simulink model "SecRwRtStFtrstIsPosChk"  (R2024b)
settings: Solver=FixedStepDiscrete  StartTime=0.0  StopTime=10.0  FixedStep=0.01  RelTol=1e-3
undefined symbols (not defined in the file or in its folder): KeSMSuSecRwStFtrstUpwdDnwdPosDelta_Val, KeSMSuSecRwStFtrstUpwdDnwdPosTolr_Val
libraries: StIsPosChkLib x9, simulink x5
settings Model: ModifiedHistory=2023.8.1 V2.0.0 CR421790 增加模式21-26  Creator=sn2xws  LastModifiedBy=sn55gm
settings SolverCC: AlgebraicLoopSolver=TrustRegion
settings DataIOCC: SaveFormat=StructureWithTime  ReturnWorkspaceOutputs=off
settings OptimizationCC: DefaultParameterBehavior=Inlined  EnhancedBackFolding=on  PassReuseOutputArgsAs=Individual arguments  ZeroExternalMemoryAtStartup=off  ZeroInternalMemoryAtStartup=off  OptimizeBlockOrder=speed  DifferentSizesBufferReuse=on  OptimizationCustomize=off  EfficientTunableParamExpr=on
settings DebuggingCC: ParameterTunabilityLossMsg=error  UnconnectedInputMsg=warning  UnconnectedOutputMsg=warning  UnconnectedLineMsg=warning  ArithmeticOperatorsInVariantConditions=warning
settings ModelReferenceCC: EnableRefExpFcnMdlSchedulingChecks=on  ModelReferenceNumInstancesAllowed=Single
settings SFSimCC: MATLABDynamicMemAlloc=off  CustomCodeUndefinedFunction=UseInterfaceOnly
settings RTWCC: Description=AUTOSAR  SystemTargetFile=autosar.tlc  GenCodeOnly=on  TemplateMakefile=ert_default_tmf  GenerateReport=on  IncludeHyperlinkInReport=on  LaunchReport=on  DataTypeReplacement=CDataTypesFixedWidth  GenerateTraceInfo=on  GenerateTraceReport=on  GenerateTraceReportSl=on  GenerateTraceReportSf=on  GenerateTraceReportEml=on  GPUComputeCapability=3.5
settings CodeAppCC: ForceParamTrailComments=on  IgnoreCustomStorageClasses=off  OperatorAnnotations=on  SimulinkDataObjDesc=on  SFDataObjDesc=on  InsertBlockDesc=on
settings STFCustomTargetCC: TargetLangStandard=C99 (ISO)  MultiwordLength=256  ParMdlRefBuildCompliant=on  CompOptLevelCompliant=on  IncludeMdlTerminateFcn=off  CombineOutputUpdateFcns=on  SuppressErrorStatus=on  ERTCustomFileBanners=on  SupportNonFinite=off  SupportComplex=off  SupportContinuousTime=off  SupportNonInlinedSFcns=off  RemoveResetFunc=on  MATLABClassNameForMDSCustomization=Simulink.SoftwareTarget.ERTCustomization  AutosarCompliant=on  UseToolchainInfoCompliant=on  LookupTableObjectStructAxisOrder=2,1,3,4,...  LUTObjectStructOrderEvenSpacing=Size,Table,Breakpoints  SystemTargetFile=autosar.tlc
settings ERTTargetCC: TargetLangStandard=C99 (ISO)  ConcurrentExecutionCompliant=off  IncludeMdlTerminateFcn=off  SuppressErrorStatus=on  SupportNonFinite=off  SupportComplex=off  ModelStepFunctionPrototypeControlCompliant=off  CPPClassGenCompliant=off  AutosarCompliant=on  LookupTableObjectStructAxisOrder=2,1,3,4,...  LUTObjectStructOrderEvenSpacing=Size,Table,Breakpoints  ERTCustomFileTemplate=example_file_process.tlc  ERTFilePackagingFormat=Compact  BooleanTrueId=TRUE  BooleanFalseId=FALSE  DynamicArrayContainerType=coder::array

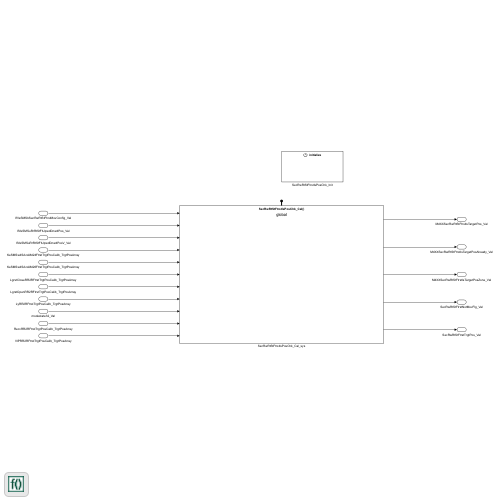
[thumbnail: Simulink's stored preview of the top-level diagram]
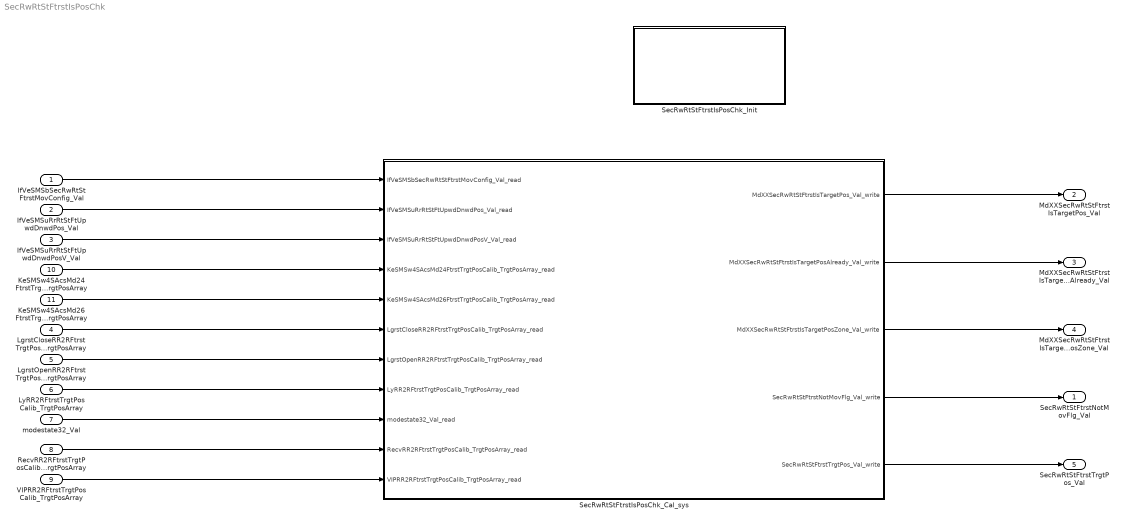
== system SecRwRtStFtrstIsPosChk ==
  IfVeSMSbSecRwRtStFtrstMovConfig_Val : Inport  OutDataTypeStr=boolean  PortDimensions=1
  IfVeSMSuRrRtStFtUpwdDnwdPos_Val : Inport  Port=2  OutDataTypeStr=uint16  PortDimensions=1
  IfVeSMSuRrRtStFtUpwdDnwdPosV_Val : Inport  Port=3  OutDataTypeStr=boolean  PortDimensions=1
  LgrstCloseRR2RFtrstTrgtPosCalib_TrgtPosArray : Inport  Description=|  Port=4  OutDataTypeStr=uint16  PortDimensions=3
      | 0:Pos
      | 1:Max
      | 2:Min
  LgrstOpenRR2RFtrstTrgtPosCalib_TrgtPosArray : Inport  Description=|  Port=5  OutDataTypeStr=uint16  PortDimensions=3
      | 0:Pos
      | 1:Max
      | 2:Min
  LyRR2RFtrstTrgtPosCalib_TrgtPosArray : Inport  Description=|  Port=6  OutDataTypeStr=uint16  PortDimensions=3
      | 0:Pos
      | 1:Max
      | 2:Min
  modestate32_Val : Inport  Port=7  OutDataTypeStr=uint32  PortDimensions=1
  RecvRR2RFtrstTrgtPosCalib_TrgtPosArray : Inport  Description=|  Port=8  OutDataTypeStr=uint16  PortDimensions=3
      | 0:Pos
      | 1:Max
      | 2:Min
  VIPRR2RFtrstTrgtPosCalib_TrgtPosArray : Inport  Description=|  Port=9  OutDataTypeStr=uint16  PortDimensions=3
      | 0:Pos
      | 1:Max
      | 2:Min
  KeSMSw4SAcsMd24FtrstTrgtPosCalib_TrgtPosArray : Inport  Description=|  Port=10  OutDataTypeStr=uint16  PortDimensions=3
      | 0:Pos
      | 1:Max
      | 2:Min
  KeSMSw4SAcsMd26FtrstTrgtPosCalib_TrgtPosArray : Inport  Description=|  Port=11  OutDataTypeStr=uint16  PortDimensions=3
      | 0:Pos
      | 1:Max
      | 2:Min
  SecRwRtStFtrstIsPosChk_Cal_sys : Subsystem
  SecRwRtStFtrstIsPosChk_Init : Subsystem
  SecRwRtStFtrstNotMovFlg_Val : Outport  OutDataTypeStr=boolean  PortDimensions=1  VectorParamsAs1DForOutWhenUnconnected=off
  MdXXSecRwRtStFtrstIsTargetPos_Val : Outport  Port=2  OutDataTypeStr=uint32  PortDimensions=1  VectorParamsAs1DForOutWhenUnconnected=off
  MdXXSecRwRtStFtrstIsTargetPosAlready_Val : Outport  Port=3  OutDataTypeStr=uint32  PortDimensions=1  VectorParamsAs1DForOutWhenUnconnected=off
  MdXXSecRwRtStFtrstIsTargetPosZone_Val : Outport  Port=4  OutDataTypeStr=uint32  PortDimensions=1  VectorParamsAs1DForOutWhenUnconnected=off
  SecRwRtStFtrstTrgtPos_Val : Outport  Port=5  OutDataTypeStr=uint16  PortDimensions=1  VectorParamsAs1DForOutWhenUnconnected=off
  wires:
  IfVeSMSbSecRwRtStFtrstMovConfig_Val/1 -> SecRwRtStFtrstIsPosChk_Cal_sys/1(IfVeSMSbSecRwRtStFtrstMovConfig_Val_read)
  IfVeSMSuRrRtStFtUpwdDnwdPos_Val/1 -> SecRwRtStFtrstIsPosChk_Cal_sys/2(IfVeSMSuRrRtStFtUpwdDnwdPos_Val_read)
  IfVeSMSuRrRtStFtUpwdDnwdPosV_Val/1 -> SecRwRtStFtrstIsPosChk_Cal_sys/3(IfVeSMSuRrRtStFtUpwdDnwdPosV_Val_read)
  LgrstCloseRR2RFtrstTrgtPosCalib_TrgtPosArray/1 -> SecRwRtStFtrstIsPosChk_Cal_sys/6(LgrstCloseRR2RFtrstTrgtPosCalib_TrgtPosArray_read)
  LgrstOpenRR2RFtrstTrgtPosCalib_TrgtPosArray/1 -> SecRwRtStFtrstIsPosChk_Cal_sys/7(LgrstOpenRR2RFtrstTrgtPosCalib_TrgtPosArray_read)
  LyRR2RFtrstTrgtPosCalib_TrgtPosArray/1 -> SecRwRtStFtrstIsPosChk_Cal_sys/8(LyRR2RFtrstTrgtPosCalib_TrgtPosArray_read)
  modestate32_Val/1 -> SecRwRtStFtrstIsPosChk_Cal_sys/9(modestate32_Val_read)
  RecvRR2RFtrstTrgtPosCalib_TrgtPosArray/1 -> SecRwRtStFtrstIsPosChk_Cal_sys/10(RecvRR2RFtrstTrgtPosCalib_TrgtPosArray_read)
  VIPRR2RFtrstTrgtPosCalib_TrgtPosArray/1 -> SecRwRtStFtrstIsPosChk_Cal_sys/11(VIPRR2RFtrstTrgtPosCalib_TrgtPosArray_read)
  SecRwRtStFtrstIsPosChk_Cal_sys/1(MdXXSecRwRtStFtrstIsTargetPos_Val_write) -> MdXXSecRwRtStFtrstIsTargetPos_Val/1
  SecRwRtStFtrstIsPosChk_Cal_sys/4(SecRwRtStFtrstNotMovFlg_Val_write) -> SecRwRtStFtrstNotMovFlg_Val/1
  SecRwRtStFtrstIsPosChk_Cal_sys/5(SecRwRtStFtrstTrgtPos_Val_write) -> SecRwRtStFtrstTrgtPos_Val/1
  KeSMSw4SAcsMd24FtrstTrgtPosCalib_TrgtPosArray/1 -> SecRwRtStFtrstIsPosChk_Cal_sys/4(KeSMSw4SAcsMd24FtrstTrgtPosCalib_TrgtPosArray_read)
  KeSMSw4SAcsMd26FtrstTrgtPosCalib_TrgtPosArray/1 -> SecRwRtStFtrstIsPosChk_Cal_sys/5(KeSMSw4SAcsMd26FtrstTrgtPosCalib_TrgtPosArray_read)
  SecRwRtStFtrstIsPosChk_Cal_sys/3(MdXXSecRwRtStFtrstIsTargetPosZone_Val_write) -> MdXXSecRwRtStFtrstIsTargetPosZone_Val/1
  SecRwRtStFtrstIsPosChk_Cal_sys/2(MdXXSecRwRtStFtrstIsTargetPosAlready_Val_write) -> MdXXSecRwRtStFtrstIsTargetPosAlready_Val/1

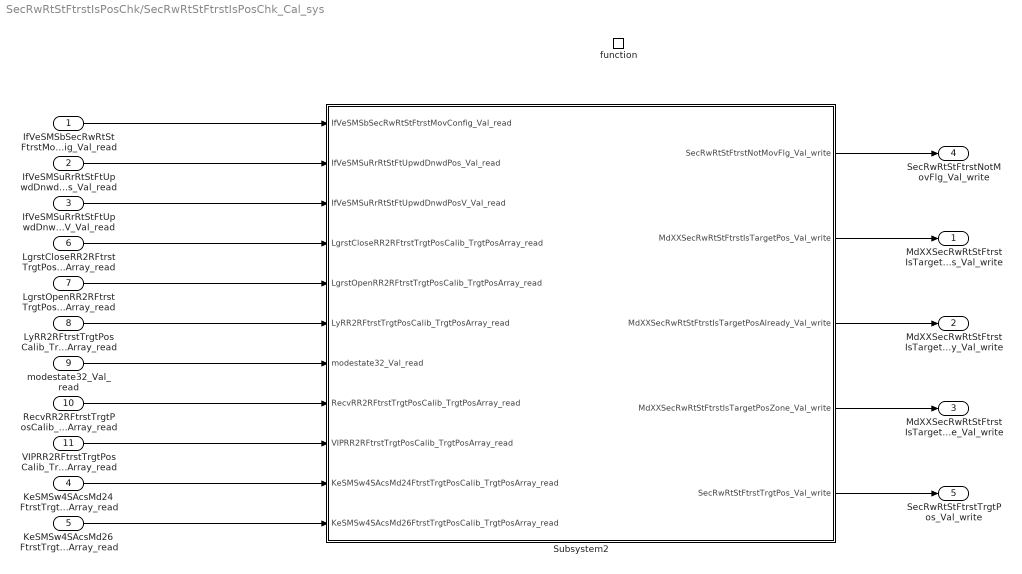
== system SecRwRtStFtrstIsPosChk/SecRwRtStFtrstIsPosChk_Cal_sys ==
  IfVeSMSbSecRwRtStFtrstMovConfig_Val_read : Inport
  IfVeSMSuRrRtStFtUpwdDnwdPos_Val_read : Inport  Port=2
  IfVeSMSuRrRtStFtUpwdDnwdPosV_Val_read : Inport  Port=3
  KeSMSw4SAcsMd24FtrstTrgtPosCalib_TrgtPosArray_read : Inport  Port=4
  KeSMSw4SAcsMd26FtrstTrgtPosCalib_TrgtPosArray_read : Inport  Port=5
  LgrstCloseRR2RFtrstTrgtPosCalib_TrgtPosArray_read : Inport  Port=6
  LgrstOpenRR2RFtrstTrgtPosCalib_TrgtPosArray_read : Inport  Port=7
  LyRR2RFtrstTrgtPosCalib_TrgtPosArray_read : Inport  Port=8
  modestate32_Val_read : Inport  Port=9
  RecvRR2RFtrstTrgtPosCalib_TrgtPosArray_read : Inport  Port=10
  VIPRR2RFtrstTrgtPosCalib_TrgtPosArray_read : Inport  Port=11
  function : TriggerPort  TriggerType=function-call  IsSimulinkFunction=on  FunctionName=SecRwRtStFtrstIsPosChk_Cal  VariantControl=(inherit)
  Subsystem2 : Subsystem
  MdXXSecRwRtStFtrstIsTargetPos_Val_write : Outport  VectorParamsAs1DForOutWhenUnconnected=off
      settings: EnsureOutportIsVirtual=on
  MdXXSecRwRtStFtrstIsTargetPosAlready_Val_write : Outport  Port=2  VectorParamsAs1DForOutWhenUnconnected=off
      settings: EnsureOutportIsVirtual=on
  MdXXSecRwRtStFtrstIsTargetPosZone_Val_write : Outport  Port=3  VectorParamsAs1DForOutWhenUnconnected=off
      settings: EnsureOutportIsVirtual=on
  SecRwRtStFtrstNotMovFlg_Val_write : Outport  Port=4  VectorParamsAs1DForOutWhenUnconnected=off
      settings: EnsureOutportIsVirtual=on
  SecRwRtStFtrstTrgtPos_Val_write : Outport  Port=5  VectorParamsAs1DForOutWhenUnconnected=off
      settings: EnsureOutportIsVirtual=on
  wires:
  LgrstCloseRR2RFtrstTrgtPosCalib_TrgtPosArray_read/1 -> Subsystem2/4(LgrstCloseRR2RFtrstTrgtPosCalib_TrgtPosArray_read)
  IfVeSMSuRrRtStFtUpwdDnwdPosV_Val_read/1 -> Subsystem2/3(IfVeSMSuRrRtStFtUpwdDnwdPosV_Val_read)
  LgrstOpenRR2RFtrstTrgtPosCalib_TrgtPosArray_read/1 -> Subsystem2/5(LgrstOpenRR2RFtrstTrgtPosCalib_TrgtPosArray_read)
  IfVeSMSuRrRtStFtUpwdDnwdPos_Val_read/1 -> Subsystem2/2(IfVeSMSuRrRtStFtUpwdDnwdPos_Val_read)
  LyRR2RFtrstTrgtPosCalib_TrgtPosArray_read/1 -> Subsystem2/6(LyRR2RFtrstTrgtPosCalib_TrgtPosArray_read)
  IfVeSMSbSecRwRtStFtrstMovConfig_Val_read/1 -> Subsystem2/1(IfVeSMSbSecRwRtStFtrstMovConfig_Val_read)
  modestate32_Val_read/1 -> Subsystem2/7(modestate32_Val_read)
  RecvRR2RFtrstTrgtPosCalib_TrgtPosArray_read/1 -> Subsystem2/8(RecvRR2RFtrstTrgtPosCalib_TrgtPosArray_read)
  VIPRR2RFtrstTrgtPosCalib_TrgtPosArray_read/1 -> Subsystem2/9(VIPRR2RFtrstTrgtPosCalib_TrgtPosArray_read)
  KeSMSw4SAcsMd24FtrstTrgtPosCalib_TrgtPosArray_read/1 -> Subsystem2/10(KeSMSw4SAcsMd24FtrstTrgtPosCalib_TrgtPosArray_read)
  KeSMSw4SAcsMd26FtrstTrgtPosCalib_TrgtPosArray_read/1 -> Subsystem2/11(KeSMSw4SAcsMd26FtrstTrgtPosCalib_TrgtPosArray_read)
  Subsystem2/1(SecRwRtStFtrstNotMovFlg_Val_write) -> SecRwRtStFtrstNotMovFlg_Val_write/1
  Subsystem2/2(MdXXSecRwRtStFtrstIsTargetPos_Val_write) -> MdXXSecRwRtStFtrstIsTargetPos_Val_write/1
  Subsystem2/3(MdXXSecRwRtStFtrstIsTargetPosAlready_Val_write) -> MdXXSecRwRtStFtrstIsTargetPosAlready_Val_write/1
  Subsystem2/4(MdXXSecRwRtStFtrstIsTargetPosZone_Val_write) -> MdXXSecRwRtStFtrstIsTargetPosZone_Val_write/1
  Subsystem2/5(SecRwRtStFtrstTrgtPos_Val_write) -> SecRwRtStFtrstTrgtPos_Val_write/1

== system SecRwRtStFtrstIsPosChk/SecRwRtStFtrstIsPosChk_Init ==
  Event Listener : EventListener  EventName=reset

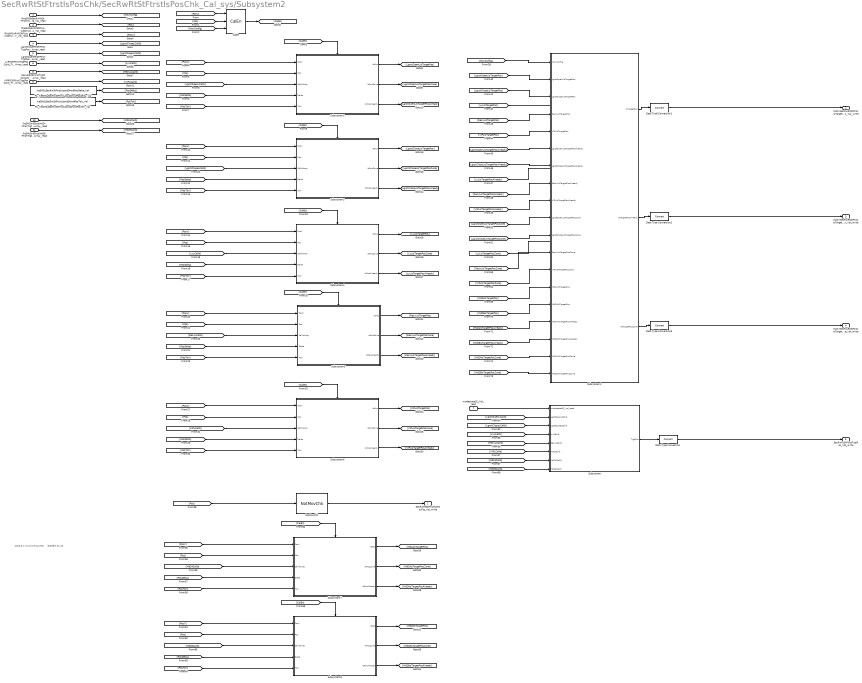
== system SecRwRtStFtrstIsPosChk/SecRwRtStFtrstIsPosChk_Cal_sys/Subsystem2 ==
  note: 2023.8.1 V2.0.0 CR421790 增加模式21-26
  IfVeSMSbSecRwRtStFtrstMovConfig_Val_read : Inport
  IfVeSMSuRrRtStFtUpwdDnwdPos_Val_read : Inport  Port=2
  IfVeSMSuRrRtStFtUpwdDnwdPosV_Val_read : Inport  Port=3
  LgrstCloseRR2RFtrstTrgtPosCalib_TrgtPosArray_read : Inport  Port=4
  LgrstOpenRR2RFtrstTrgtPosCalib_TrgtPosArray_read : Inport  Port=5
  LyRR2RFtrstTrgtPosCalib_TrgtPosArray_read : Inport  Port=6
  modestate32_Val_read : Inport  Port=7
  RecvRR2RFtrstTrgtPosCalib_TrgtPosArray_read : Inport  Port=8
  VIPRR2RFtrstTrgtPosCalib_TrgtPosArray_read : Inport  Port=9
  KeSMSw4SAcsMd24FtrstTrgtPosCalib_TrgtPosArray_read : Inport  Port=10
  KeSMSw4SAcsMd26FtrstTrgtPosCalib_TrgtPosArray_read : Inport  Port=11
  CalEn : StIsPosChkLib/CalEn  SystemSampleTime=-1  VariantActivationTime=update diagram  AllowFlexibleInterface=on  Latency=0  AutoFrameSizeCalculation=off
  Data Type Conversion{,1..3} (4 alike) : DataTypeConversion  SaturateOnIntegerOverflow=off  RndMeth=Floor
  NotMovChk : StIsPosChkLib/NotMovChk  SystemSampleTime=-1  VariantActivationTime=update diagram  AllowFlexibleInterface=on  Latency=0  AutoFrameSizeCalculation=off
  PA_KeSMSuSecRwStFtrstUpwdDnwdPosDelta_Val : Constant  Value=KeSMSuSecRwStFtrstUpwdDnwdPosDelta_Val
  PA_KeSMSuSecRwStFtrstUpwdDnwdPosTolr_Val : Constant  Value=KeSMSuSecRwStFtrstUpwdDnwdPosTolr_Val
  Subsystem : Subsystem
  Subsystem1 : Subsystem
  Subsystem2 : Subsystem
  Subsystem3 : Subsystem
  Subsystem4 : Subsystem
  Subsystem5 : Subsystem
  Subsystem6 : Subsystem
  Subsystem7 : Subsystem
  Subsystem8 : Subsystem
  SecRwRtStFtrstNotMovFlg_Val_write : Outport  VectorParamsAs1DForOutWhenUnconnected=off
      settings: EnsureOutportIsVirtual=on
  MdXXSecRwRtStFtrstIsTargetPos_Val_write : Outport  Port=2  VectorParamsAs1DForOutWhenUnconnected=off
      settings: EnsureOutportIsVirtual=on
  MdXXSecRwRtStFtrstIsTargetPosAlready_Val_write : Outport  Port=3  VectorParamsAs1DForOutWhenUnconnected=off
      settings: EnsureOutportIsVirtual=on
  MdXXSecRwRtStFtrstIsTargetPosZone_Val_write : Outport  Port=4  VectorParamsAs1DForOutWhenUnconnected=off
      settings: EnsureOutportIsVirtual=on
  SecRwRtStFtrstTrgtPos_Val_write : Outport  Port=5  VectorParamsAs1DForOutWhenUnconnected=off
      settings: EnsureOutportIsVirtual=on
  wires:
  VIPRR2RFtrstTrgtPosCalib_TrgtPosArray_read/1 -> [VIPLCalib]
  Subsystem2/3(IsPosAlready) -> [LgrstOpenLIsTargetPosAlready]
  IfVeSMSuRrRtStFtUpwdDnwdPosV_Val_read/1 -> [PosV]
  Subsystem4/1(IsPos) -> [LyLIsTargetPos]
  IfVeSMSbSecRwRtStFtrstMovConfig_Val_read/1 -> [MovConfig]
  [CalEn] -> Subsystem5/Enable
  LgrstCloseRR2RFtrstTrgtPosCalib_TrgtPosArray_read/1 -> [LgrstCloseLCalib]
  [Pos] -> Subsystem5/2(Pos)
  IfVeSMSuRrRtStFtUpwdDnwdPos_Val_read/1 -> [Pos]
  [RecvLIsTargetPos] -> Subsystem1/4(RecvLIsTargetPos)
  [LgrstCloseLCalib] -> Subsystem/3(LgrstCloseLCalib)
  [LyLCalib] -> Subsystem/4(LyLCalib)
  [Pos] -> NotMovChk/1
  [Pos] -> Subsystem4/2(Pos)
  [PosTolr] -> Subsystem3/5(Tolr)
  PA_KeSMSuSecRwStFtrstUpwdDnwdPosTolr_Val/1 -> [PosTolr]
  [LgrstCloseLIsTargetPos] -> Subsystem1/3(LgrstCloseLIsTargetPos)
  Subsystem6/2(IsPosZone) -> [VIPLIsTargetPosZone]
  [LgrstOpenLCalib] -> Subsystem/2(LgrstOpenLCalib)
  [RecvLIsTargetPosAlready] -> Subsystem1/8(RecvLIsTargetPosAlready)
  [PosDelta] -> Subsystem4/4(Delta)
  Subsystem1/1(IsTargetPos) -> Data Type Conversion1/1
  PA_KeSMSuSecRwStFtrstUpwdDnwdPosDelta_Val/1 -> [PosDelta]
  Subsystem1/2(IsTargetPosAlready) -> Data Type Conversion2/1
  Subsystem6/3(IsPosAlready) -> [VIPLIsTargetPosAlready]
  [PosV] -> CalEn/1
  RecvRR2RFtrstTrgtPosCalib_TrgtPosArray_read/1 -> [RecvLCalib]
  [LgrstCloseLIsTargetPosZone] -> Subsystem1/11(LgrstCloseLIsTargetPosZone)
  [PosV] -> Subsystem2/1(PosV)
  [PosV] -> Subsystem6/1(PosV)
  [PosDelta] -> Subsystem3/4(Delta)
  LyRR2RFtrstTrgtPosCalib_TrgtPosArray_read/1 -> [LyLCalib]
  [RecvLIsTargetPosZone] -> Subsystem1/12(RecvLIsTargetPosZone)
  [LyLIsTargetPos] -> ?
  Data Type Conversion/1 -> SecRwRtStFtrstTrgtPos_Val_write/1
  [LyLIsTargetPosAlready] -> ?
  [MovConfig] -> Subsystem1/1(MovConfig)
  Data Type Conversion3/1 -> MdXXSecRwRtStFtrstIsTargetPosZone_Val_write/1
  [PosDelta] -> Subsystem6/4(Delta)
  [VIPLIsTargetPos] -> Subsystem1/5(VIPLIsTargetPos)
  [VIPLIsTargetPosAlready] -> Subsystem1/9(VIPLIsTargetPosAlready)
  Subsystem5/3(IsPosAlready) -> [RecvLIsTargetPosAlready]
  Subsystem4/2(IsPosZone) -> [LyLIsTargetPosZone]
  [RecvLCalib] -> Subsystem/5(RecvLCalib)
  Subsystem1/3(IsTargetPosZone) -> Data Type Conversion3/1
  Subsystem6/1(IsPos) -> [VIPLIsTargetPos]
  [VIPLIsTargetPosZone] -> Subsystem1/13(VIPLIsTargetPosZone)
  [LgrstOpenLIsTargetPos] -> Subsystem1/2(LgrstOpenLIsTargetPos)
  Subsystem/1(TrgtPos) -> Data Type Conversion/1
  [PosDelta] -> Subsystem5/4(Delta)
  [CalEn] -> Subsystem4/Enable
  Data Type Conversion2/1 -> MdXXSecRwRtStFtrstIsTargetPosAlready_Val_write/1
  Data Type Conversion1/1 -> MdXXSecRwRtStFtrstIsTargetPos_Val_write/1
  [Pos] -> Subsystem2/2(Pos)
  [CalEn] -> Subsystem3/Enable
  [LyLCalib] -> Subsystem4/3(CalibArray)
  [CalEn] -> Subsystem6/Enable
  [CalEn] -> Subsystem2/Enable
  [LgrstOpenLIsTargetPosAlready] -> Subsystem1/6(LgrstOpenLIsTargetPosAlready)
  [PosTolr] -> Subsystem2/5(Tolr)
  [PosV] -> Subsystem5/1(PosV)
  [MovConfig] -> CalEn/3
  Subsystem2/1(IsPos) -> [LgrstOpenLIsTargetPos]
  LgrstOpenRR2RFtrstTrgtPosCalib_TrgtPosArray_read/1 -> [LgrstOpenLCalib]
  Subsystem3/2(IsPosZone) -> [LgrstCloseLIsTargetPosZone]
  [Pos] -> CalEn/2
  [PosTolr] -> Subsystem4/5(Tolr)
  [LgrstOpenLIsTargetPosZone] -> Subsystem1/10(LgrstOpenLIsTargetPosZone)
  [LyLIsTargetPosZone] -> ?
  [PosDelta] -> Subsystem2/4(Delta)
  [LgrstCloseLIsTargetPosAlready] -> Subsystem1/7(LgrstCloseLIsTargetPosAlready)
  Subsystem3/1(IsPos) -> [LgrstCloseLIsTargetPos]
  [RecvLCalib] -> Subsystem5/3(CalibArray)
  [Pos] -> Subsystem6/2(Pos)
  [PosV] -> Subsystem3/1(PosV)
  Subsystem4/3(IsPosAlready) -> [LyLIsTargetPosAlready]
  [PosTolr] -> Subsystem6/5(Tolr)
  CalEn/1 -> [CalEn]
  [PosTolr] -> Subsystem5/5(Tolr)
  [VIPLCalib] -> Subsystem6/3(CalibArray)
  Subsystem2/2(IsPosZone) -> [LgrstOpenLIsTargetPosZone]
  Subsystem5/2(IsPosZone) -> [RecvLIsTargetPosZone]
  [PosV] -> Subsystem4/1(PosV)
  [Pos] -> Subsystem3/2(Pos)
  Subsystem3/3(IsPosAlready) -> [LgrstCloseLIsTargetPosAlready]
  Subsystem5/1(IsPos) -> [RecvLIsTargetPos]
  modestate32_Val_read/1 -> Subsystem/1(modestate32_Val_read)
  [VIPLCalib] -> Subsystem/6(VIPLCalib)
  NotMovChk/1 -> SecRwRtStFtrstNotMovFlg_Val_write/1
  KeSMSw4SAcsMd24FtrstTrgtPosCalib_TrgtPosArray_read/1 -> [Md24Calib]
  KeSMSw4SAcsMd26FtrstTrgtPosCalib_TrgtPosArray_read/1 -> [Md26Calib]
  [Md24Calib] -> Subsystem7/3(CalibArray)
  [PosTolr] -> Subsystem7/5(Tolr)
  [Pos] -> Subsystem7/2(Pos)
  [CalEn] -> Subsystem7/Enable
  Subsystem7/1(IsPos) -> [Md24IsTargetPos]
  [PosDelta] -> Subsystem7/4(Delta)
  [PosV] -> Subsystem7/1(PosV)
  Subsystem7/3(IsPosAlready) -> [Md24IsTargetPosAlready]
  Subsystem7/2(IsPosZone) -> [Md24IsTargetPosZone]
  Subsystem8/2(IsPosZone) -> [Md26IsTargetPosZone]
  Subsystem8/3(IsPosAlready) -> [Md26IsTargetPosAlready]
  [PosV] -> Subsystem8/1(PosV)
  [PosDelta] -> Subsystem8/4(Delta)
  Subsystem8/1(IsPos) -> [Md26IsTargetPos]
  [CalEn] -> Subsystem8/Enable
  [Pos] -> Subsystem8/2(Pos)
  [PosTolr] -> Subsystem8/5(Tolr)
  [Md26Calib] -> Subsystem8/3(CalibArray)
  [Md24Calib] -> Subsystem/7(Md24Calib)
  [Md26Calib] -> Subsystem/8(Md26Calib)
  [Md24IsTargetPos] -> Subsystem1/14(Md24IsTargetPos)
  [Md26IsTargetPos] -> Subsystem1/15(Md26IsTargetPos)
  [Md24IsTargetPosAlready] -> Subsystem1/16(Md24IsTargetPosAlready)
  [Md26IsTargetPosAlready] -> Subsystem1/17(Md26IsTargetPosAlready)
  [Md26IsTargetPosZone] -> Subsystem1/19(Md26IsTargetPosZone)
  [Md24IsTargetPosZone] -> Subsystem1/18(Md24IsTargetPosZone)
  [LgrstOpenLCalib] -> Subsystem2/3(CalibArray)
  [LgrstCloseLCalib] -> Subsystem3/3(CalibArray)

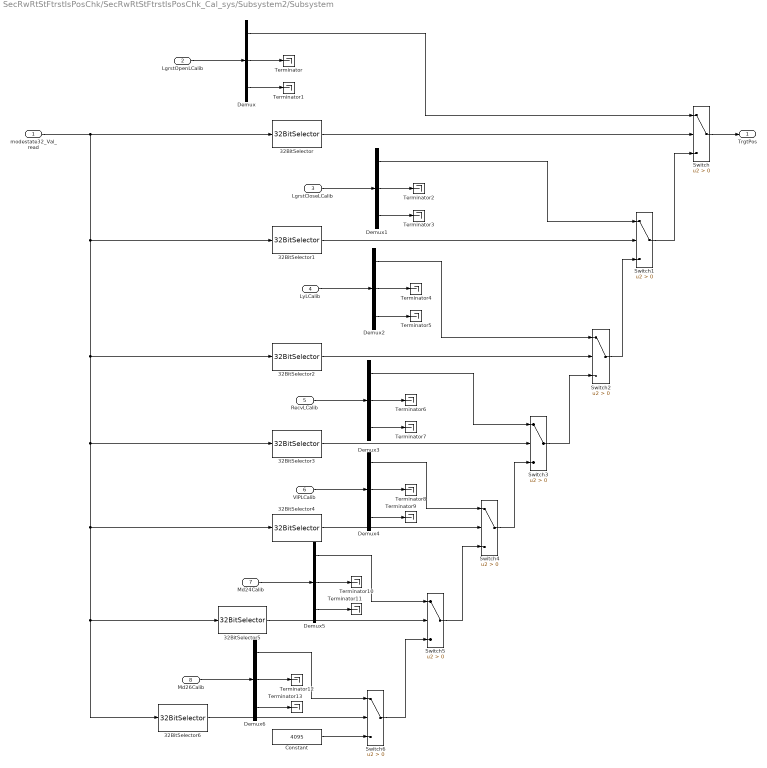
== system SecRwRtStFtrstIsPosChk/SecRwRtStFtrstIsPosChk_Cal_sys/Subsystem2/Subsystem ==
  modestate32_Val_read : Inport
  LgrstOpenLCalib : Inport  Port=2
  LgrstCloseLCalib : Inport  Port=3
  LyLCalib : Inport  Port=4
  RecvLCalib : Inport  Port=5
  VIPLCalib : Inport  Port=6
  Md24Calib : Inport  Port=7
  Md26Calib : Inport  Port=8
  32BitSelector : StIsPosChkLib/32BitSelector  BitNum=17
  32BitSelector1 : StIsPosChkLib/32BitSelector  BitNum=18
  32BitSelector2 : StIsPosChkLib/32BitSelector  BitNum=14
  32BitSelector3 : StIsPosChkLib/32BitSelector  BitNum=12
  32BitSelector4 : StIsPosChkLib/32BitSelector  BitNum=11
  32BitSelector5 : StIsPosChkLib/32BitSelector  BitNum=23
  32BitSelector6 : StIsPosChkLib/32BitSelector  BitNum=25
  Constant : Constant  Value=4095  OutDataTypeStr=uint16
  Demux{,1..6} (7 alike) : Demux  Outputs=3
  Switch{,1..6} (7 alike) : Switch  Criteria=u2 > Threshold  SaturateOnIntegerOverflow=off  InputSameDT=off
  Terminator{,1..13} (14 alike) : Terminator
  TrgtPos : Outport  VectorParamsAs1DForOutWhenUnconnected=off
      settings: EnsureOutportIsVirtual=on
  wires:
  32BitSelector/1 -> Switch/2
  modestate32_Val_read/1 -> 32BitSelector/1, 32BitSelector1/1, 32BitSelector2/1, 32BitSelector3/1, 32BitSelector6/1, 32BitSelector5/1, 32BitSelector4/1
  Demux/1 -> Switch/1
  Demux/3 -> Terminator1/1
  Demux/2 -> Terminator/1
  LgrstOpenLCalib/1 -> Demux/1
  LgrstCloseLCalib/1 -> Demux1/1
  Demux1/2 -> Terminator2/1
  Demux1/3 -> Terminator3/1
  Demux1/1 -> Switch1/1
  Switch/1 -> TrgtPos/1
  Switch1/1 -> Switch/3
  32BitSelector1/1 -> Switch1/2
  Switch2/1 -> Switch1/3
  Switch3/1 -> Switch2/3
  Switch4/1 -> Switch3/3
  32BitSelector2/1 -> Switch2/2
  32BitSelector3/1 -> Switch3/2
  32BitSelector4/1 -> Switch4/2
  Demux2/1 -> Switch2/1
  Demux2/3 -> Terminator5/1
  Demux2/2 -> Terminator4/1
  LyLCalib/1 -> Demux2/1
  RecvLCalib/1 -> Demux3/1
  Demux3/2 -> Terminator6/1
  Demux3/3 -> Terminator7/1
  Demux3/1 -> Switch3/1
  Demux4/1 -> Switch4/1
  Demux4/3 -> Terminator9/1
  Demux4/2 -> Terminator8/1
  VIPLCalib/1 -> Demux4/1
  Md24Calib/1 -> Demux5/1
  Demux5/2 -> Terminator10/1
  Demux5/3 -> Terminator11/1
  Demux5/1 -> Switch5/1
  32BitSelector5/1 -> Switch5/2
  Switch5/1 -> Switch4/3
  Switch6/1 -> Switch5/3
  32BitSelector6/1 -> Switch6/2
  Demux6/1 -> Switch6/1
  Demux6/3 -> Terminator13/1
  Demux6/2 -> Terminator12/1
  Md26Calib/1 -> Demux6/1
  Constant/1 -> Switch6/3

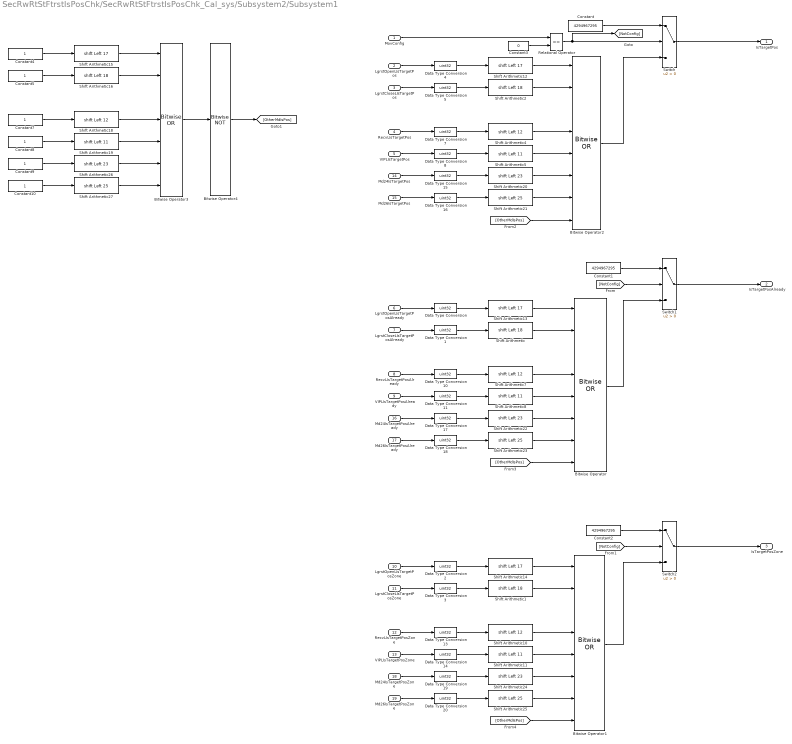
== system SecRwRtStFtrstIsPosChk/SecRwRtStFtrstIsPosChk_Cal_sys/Subsystem2/Subsystem1 ==
  MovConfig : Inport
  LgrstOpenLIsTargetPos : Inport  Port=2
  LgrstCloseLIsTargetPos : Inport  Port=3
  RecvLIsTargetPos : Inport  Port=4
  VIPLIsTargetPos : Inport  Port=5
  LgrstOpenLIsTargetPosAlready : Inport  Port=6
  LgrstCloseLIsTargetPosAlready : Inport  Port=7
  RecvLIsTargetPosAlready : Inport  Port=8
  VIPLIsTargetPosAlready : Inport  Port=9
  LgrstOpenLIsTargetPosZone : Inport  Port=10
  LgrstCloseLIsTargetPosZone : Inport  Port=11
  RecvLIsTargetPosZone : Inport  Port=12
  VIPLIsTargetPosZone : Inport  Port=13
  Md24IsTargetPos : Inport  Port=14
  Md26IsTargetPos : Inport  Port=15
  Md24IsTargetPosAlready : Inport  Port=16
  Md26IsTargetPosAlready : Inport  Port=17
  Md24IsTargetPosZone : Inport  Port=18
  Md26IsTargetPosZone : Inport  Port=19
  Bitwise Operator : simulink/Logic and Bit Operations/Bitwise Operator  logicop=OR  UseBitMask=off  NumInputPorts=8  BitMask=bin2dec('11011001')  BitMaskRealWorld=Stored Integer
  Bitwise Operator1 : simulink/Logic and Bit Operations/Bitwise Operator  logicop=OR  UseBitMask=off  NumInputPorts=8  BitMask=bin2dec('11011001')  BitMaskRealWorld=Stored Integer
  Bitwise Operator2 : simulink/Logic and Bit Operations/Bitwise Operator  logicop=OR  UseBitMask=off  NumInputPorts=8  BitMask=bin2dec('11011001')  BitMaskRealWorld=Stored Integer
  Bitwise Operator3 : simulink/Logic and Bit Operations/Bitwise Operator  logicop=OR  UseBitMask=off  NumInputPorts=7  BitMask=bin2dec('11011001')  BitMaskRealWorld=Stored Integer
  Bitwise Operator4 : simulink/Logic and Bit Operations/Bitwise Operator  logicop=NOT  UseBitMask=off  BitMask=bin2dec('11011001')  BitMaskRealWorld=Stored Integer
  Constant : Constant  Value=4294967295  OutDataTypeStr=uint32
  Constant1 : Constant  Value=4294967295  OutDataTypeStr=uint32
  Constant{4..5,7..10} (6 alike) : Constant  OutDataTypeStr=uint32
  Constant2 : Constant  Value=4294967295  OutDataTypeStr=uint32
  Constant3 : Constant  Value=0  OutDataTypeStr=uint8
  Data Type Conversion{,1..5,7..8,10..11,13..20} (18 alike) : DataTypeConversion  OutDataTypeStr=uint32  SaturateOnIntegerOverflow=off  RndMeth=Floor
  Relational Operator : RelationalOperator  Operator===  OutDataTypeStr=boolean  RndMeth=Simplest  InputSameDT=off
  Shift Arithmetic{,1..2,16} (4 alike) : ArithShift  BitShiftNumber=18  BitShiftDirection=Left
  Shift Arithmetic{4,7,10,18} (4 alike) : ArithShift  BitShiftNumber=12  BitShiftDirection=Left
  Shift Arithmetic{5,8,11,19} (4 alike) : ArithShift  BitShiftNumber=11  BitShiftDirection=Left
  Shift Arithmetic{12..15} (4 alike) : ArithShift  BitShiftNumber=17  BitShiftDirection=Left
  Shift Arithmetic{20,22,24,26} (4 alike) : ArithShift  BitShiftNumber=23  BitShiftDirection=Left
  Shift Arithmetic{21,23,25,27} (4 alike) : ArithShift  BitShiftNumber=25  BitShiftDirection=Left
  Switch : Switch  Criteria=u2 > Threshold  SaturateOnIntegerOverflow=off  InputSameDT=off
  Switch1 : Switch  Criteria=u2 > Threshold  SaturateOnIntegerOverflow=off  InputSameDT=off
  Switch2 : Switch  Criteria=u2 > Threshold  SaturateOnIntegerOverflow=off  InputSameDT=off
  IsTargetPos : Outport  VectorParamsAs1DForOutWhenUnconnected=off
      settings: EnsureOutportIsVirtual=on
  IsTargetPosAlready : Outport  Port=2  VectorParamsAs1DForOutWhenUnconnected=off
      settings: EnsureOutportIsVirtual=on
  IsTargetPosZone : Outport  Port=3  VectorParamsAs1DForOutWhenUnconnected=off
      settings: EnsureOutportIsVirtual=on
  wires:
  Constant3/1 -> Relational Operator/2
  Constant/1 -> Switch/1
  Relational Operator/1 -> [NotConfig], Switch/2
  MovConfig/1 -> Relational Operator/1
  Switch/1 -> IsTargetPos/1
  [NotConfig] -> Switch1/2
  Constant1/1 -> Switch1/1
  Switch1/1 -> IsTargetPosAlready/1
  Switch2/1 -> IsTargetPosZone/1
  Constant2/1 -> Switch2/1
  [NotConfig] -> Switch2/2
  Data Type Conversion1/1 -> Shift Arithmetic/1
  Data Type Conversion/1 -> Shift Arithmetic13/1
  Shift Arithmetic/1 -> Bitwise Operator/2
  Shift Arithmetic1/1 -> Bitwise Operator1/2
  Data Type Conversion2/1 -> Shift Arithmetic14/1
  Data Type Conversion3/1 -> Shift Arithmetic1/1
  Bitwise Operator1/1 -> Switch2/3
  Bitwise Operator/1 -> Switch1/3
  Shift Arithmetic2/1 -> Bitwise Operator2/2
  Data Type Conversion4/1 -> Shift Arithmetic12/1
  Data Type Conversion5/1 -> Shift Arithmetic2/1
  Bitwise Operator2/1 -> Switch/3
  LgrstOpenLIsTargetPos/1 -> Data Type Conversion4/1
  LgrstCloseLIsTargetPos/1 -> Data Type Conversion5/1
  LgrstCloseLIsTargetPosZone/1 -> Data Type Conversion3/1
  LgrstOpenLIsTargetPosZone/1 -> Data Type Conversion2/1
  LgrstCloseLIsTargetPosAlready/1 -> Data Type Conversion1/1
  LgrstOpenLIsTargetPosAlready/1 -> Data Type Conversion/1
  Shift Arithmetic4/1 -> Bitwise Operator2/4
  Shift Arithmetic5/1 -> Bitwise Operator2/5
  Data Type Conversion7/1 -> Shift Arithmetic4/1
  Data Type Conversion8/1 -> Shift Arithmetic5/1
  RecvLIsTargetPos/1 -> Data Type Conversion7/1
  VIPLIsTargetPos/1 -> Data Type Conversion8/1
  VIPLIsTargetPosAlready/1 -> Data Type Conversion11/1
  RecvLIsTargetPosAlready/1 -> Data Type Conversion10/1
  Data Type Conversion11/1 -> Shift Arithmetic8/1
  Data Type Conversion10/1 -> Shift Arithmetic7/1
  Shift Arithmetic8/1 -> Bitwise Operator/5
  Shift Arithmetic7/1 -> Bitwise Operator/4
  Data Type Conversion14/1 -> Shift Arithmetic11/1
  Data Type Conversion13/1 -> Shift Arithmetic10/1
  VIPLIsTargetPosZone/1 -> Data Type Conversion14/1
  Shift Arithmetic10/1 -> Bitwise Operator1/4
  RecvLIsTargetPosZone/1 -> Data Type Conversion13/1
  Shift Arithmetic11/1 -> Bitwise Operator1/5
  Shift Arithmetic12/1 -> Bitwise Operator2/1
  Shift Arithmetic13/1 -> Bitwise Operator/1
  Shift Arithmetic14/1 -> Bitwise Operator1/1
  Shift Arithmetic15/1 -> Bitwise Operator3/1
  Constant8/1 -> Shift Arithmetic19/1
  Constant7/1 -> Shift Arithmetic18/1
  Shift Arithmetic19/1 -> Bitwise Operator3/5
  Shift Arithmetic18/1 -> Bitwise Operator3/4
  Constant5/1 -> Shift Arithmetic16/1
  Constant4/1 -> Shift Arithmetic15/1
  Shift Arithmetic16/1 -> Bitwise Operator3/2
  Bitwise Operator3/1 -> Bitwise Operator4/1
  Bitwise Operator4/1 -> [OtherMdIsPos]
  [OtherMdIsPos] -> Bitwise Operator2/8
  Md24IsTargetPos/1 -> Data Type Conversion15/1
  Data Type Conversion15/1 -> Shift Arithmetic20/1
  Shift Arithmetic20/1 -> Bitwise Operator2/6
  Shift Arithmetic21/1 -> Bitwise Operator2/7
  Data Type Conversion16/1 -> Shift Arithmetic21/1
  Md26IsTargetPos/1 -> Data Type Conversion16/1
  [OtherMdIsPos] -> Bitwise Operator/8
  Shift Arithmetic22/1 -> Bitwise Operator/6
  Data Type Conversion17/1 -> Shift Arithmetic22/1
  Md24IsTargetPosAlready/1 -> Data Type Conversion17/1
  Md26IsTargetPosAlready/1 -> Data Type Conversion18/1
  Data Type Conversion18/1 -> Shift Arithmetic23/1
  Shift Arithmetic23/1 -> Bitwise Operator/7
  [OtherMdIsPos] -> Bitwise Operator1/8
  Shift Arithmetic24/1 -> Bitwise Operator1/6
  Md24IsTargetPosZone/1 -> Data Type Conversion19/1
  Data Type Conversion19/1 -> Shift Arithmetic24/1
  Data Type Conversion20/1 -> Shift Arithmetic25/1
  Md26IsTargetPosZone/1 -> Data Type Conversion20/1
  Shift Arithmetic25/1 -> Bitwise Operator1/7
  Shift Arithmetic26/1 -> Bitwise Operator3/6
  Constant9/1 -> Shift Arithmetic26/1
  Constant10/1 -> Shift Arithmetic27/1
  Shift Arithmetic27/1 -> Bitwise Operator3/7

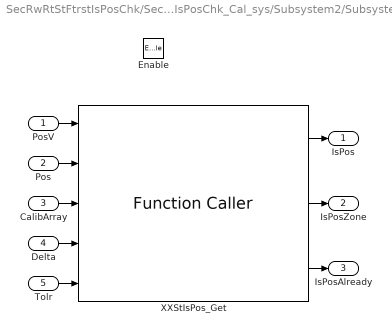
== system SecRwRtStFtrstIsPosChk/SecRwRtStFtrstIsPosChk_Cal_sys/Subsystem2/Subsystem2 ==
  PosV : Inport
  Pos : Inport  Port=2
  CalibArray : Inport  Port=3
  Delta : Inport  Port=4
  Tolr : Inport  Port=5
  Enable : EnablePort
  XXStIsPos_Get : FunctionCaller  FunctionPrototype=[IsPos,IsPosZone,IsPosAlready] = XXStIsPos_Get(PosV,Pos,CalibArray,Delta,Tolr)  InputArgumentSpecifications=boolean(true), uint16(1), uint16([1;1;1]), uint16(1), uint16(1)  OutputArgumentSpecifications=boolean(true), boolean(true), boolean(true)
  IsPos : Outport  VectorParamsAs1DForOutWhenUnconnected=off
  IsPosZone : Outport  Port=2  VectorParamsAs1DForOutWhenUnconnected=off
  IsPosAlready : Outport  Port=3  VectorParamsAs1DForOutWhenUnconnected=off
  wires:
  Delta/1 -> XXStIsPos_Get/4
  Tolr/1 -> XXStIsPos_Get/5
  XXStIsPos_Get/3 -> IsPosAlready/1
  XXStIsPos_Get/2 -> IsPosZone/1
  PosV/1 -> XXStIsPos_Get/1
  Pos/1 -> XXStIsPos_Get/2
  CalibArray/1 -> XXStIsPos_Get/3
  XXStIsPos_Get/1 -> IsPos/1

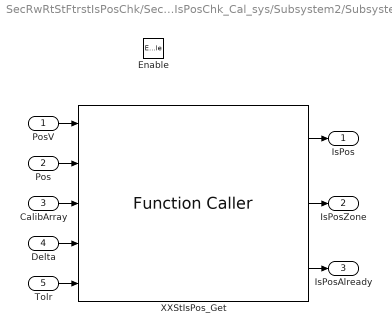
== system SecRwRtStFtrstIsPosChk/SecRwRtStFtrstIsPosChk_Cal_sys/Subsystem2/Subsystem3 ==
  PosV : Inport
  Pos : Inport  Port=2
  CalibArray : Inport  Port=3
  Delta : Inport  Port=4
  Tolr : Inport  Port=5
  Enable : EnablePort
  XXStIsPos_Get : FunctionCaller  FunctionPrototype=[IsPos,IsPosZone,IsPosAlready] = XXStIsPos_Get(PosV,Pos,CalibArray,Delta,Tolr)  InputArgumentSpecifications=boolean(true), uint16(1), uint16([1;1;1]), uint16(1), uint16(1)  OutputArgumentSpecifications=boolean(true), boolean(true), boolean(true)
  IsPos : Outport  VectorParamsAs1DForOutWhenUnconnected=off
  IsPosZone : Outport  Port=2  VectorParamsAs1DForOutWhenUnconnected=off
  IsPosAlready : Outport  Port=3  VectorParamsAs1DForOutWhenUnconnected=off
  wires:
  XXStIsPos_Get/1 -> IsPos/1
  CalibArray/1 -> XXStIsPos_Get/3
  Pos/1 -> XXStIsPos_Get/2
  PosV/1 -> XXStIsPos_Get/1
  XXStIsPos_Get/2 -> IsPosZone/1
  XXStIsPos_Get/3 -> IsPosAlready/1
  Tolr/1 -> XXStIsPos_Get/5
  Delta/1 -> XXStIsPos_Get/4

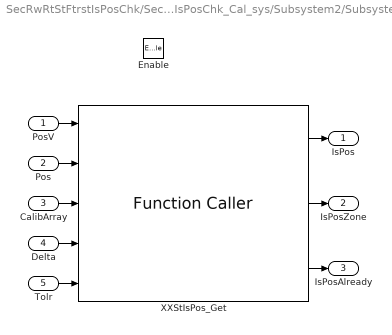
== system SecRwRtStFtrstIsPosChk/SecRwRtStFtrstIsPosChk_Cal_sys/Subsystem2/Subsystem4 ==
  PosV : Inport
  Pos : Inport  Port=2
  CalibArray : Inport  Port=3
  Delta : Inport  Port=4
  Tolr : Inport  Port=5
  Enable : EnablePort
  XXStIsPos_Get : FunctionCaller  FunctionPrototype=[IsPos,IsPosZone,IsPosAlready] = XXStIsPos_Get(PosV,Pos,CalibArray,Delta,Tolr)  InputArgumentSpecifications=boolean(true), uint16(1), uint16([1;1;1]), uint16(1), uint16(1)  OutputArgumentSpecifications=boolean(true), boolean(true), boolean(true)
  IsPos : Outport  VectorParamsAs1DForOutWhenUnconnected=off
  IsPosZone : Outport  Port=2  VectorParamsAs1DForOutWhenUnconnected=off
  IsPosAlready : Outport  Port=3  VectorParamsAs1DForOutWhenUnconnected=off
  wires:
  Delta/1 -> XXStIsPos_Get/4
  Tolr/1 -> XXStIsPos_Get/5
  XXStIsPos_Get/3 -> IsPosAlready/1
  XXStIsPos_Get/2 -> IsPosZone/1
  PosV/1 -> XXStIsPos_Get/1
  Pos/1 -> XXStIsPos_Get/2
  CalibArray/1 -> XXStIsPos_Get/3
  XXStIsPos_Get/1 -> IsPos/1

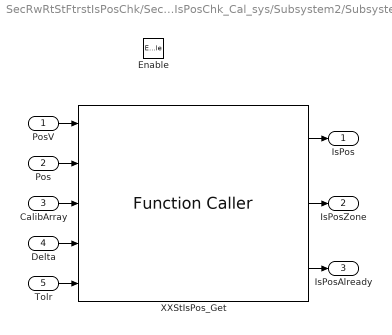
== system SecRwRtStFtrstIsPosChk/SecRwRtStFtrstIsPosChk_Cal_sys/Subsystem2/Subsystem5 ==
  PosV : Inport
  Pos : Inport  Port=2
  CalibArray : Inport  Port=3
  Delta : Inport  Port=4
  Tolr : Inport  Port=5
  Enable : EnablePort
  XXStIsPos_Get : FunctionCaller  FunctionPrototype=[IsPos,IsPosZone,IsPosAlready] = XXStIsPos_Get(PosV,Pos,CalibArray,Delta,Tolr)  InputArgumentSpecifications=boolean(true), uint16(1), uint16([1;1;1]), uint16(1), uint16(1)  OutputArgumentSpecifications=boolean(true), boolean(true), boolean(true)
  IsPos : Outport  VectorParamsAs1DForOutWhenUnconnected=off
  IsPosZone : Outport  Port=2  VectorParamsAs1DForOutWhenUnconnected=off
  IsPosAlready : Outport  Port=3  VectorParamsAs1DForOutWhenUnconnected=off
  wires:
  XXStIsPos_Get/1 -> IsPos/1
  CalibArray/1 -> XXStIsPos_Get/3
  Pos/1 -> XXStIsPos_Get/2
  PosV/1 -> XXStIsPos_Get/1
  XXStIsPos_Get/2 -> IsPosZone/1
  XXStIsPos_Get/3 -> IsPosAlready/1
  Tolr/1 -> XXStIsPos_Get/5
  Delta/1 -> XXStIsPos_Get/4

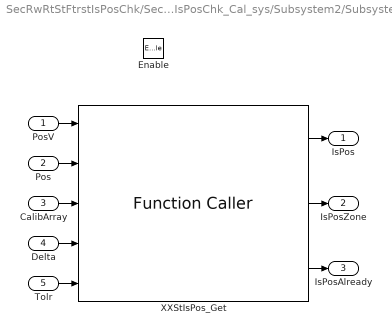
== system SecRwRtStFtrstIsPosChk/SecRwRtStFtrstIsPosChk_Cal_sys/Subsystem2/Subsystem6 ==
  PosV : Inport
  Pos : Inport  Port=2
  CalibArray : Inport  Port=3
  Delta : Inport  Port=4
  Tolr : Inport  Port=5
  Enable : EnablePort
  XXStIsPos_Get : FunctionCaller  FunctionPrototype=[IsPos,IsPosZone,IsPosAlready] = XXStIsPos_Get(PosV,Pos,CalibArray,Delta,Tolr)  InputArgumentSpecifications=boolean(true), uint16(1), uint16([1;1;1]), uint16(1), uint16(1)  OutputArgumentSpecifications=boolean(true), boolean(true), boolean(true)
  IsPos : Outport  VectorParamsAs1DForOutWhenUnconnected=off
  IsPosZone : Outport  Port=2  VectorParamsAs1DForOutWhenUnconnected=off
  IsPosAlready : Outport  Port=3  VectorParamsAs1DForOutWhenUnconnected=off
  wires:
  Delta/1 -> XXStIsPos_Get/4
  Tolr/1 -> XXStIsPos_Get/5
  XXStIsPos_Get/3 -> IsPosAlready/1
  XXStIsPos_Get/2 -> IsPosZone/1
  PosV/1 -> XXStIsPos_Get/1
  Pos/1 -> XXStIsPos_Get/2
  CalibArray/1 -> XXStIsPos_Get/3
  XXStIsPos_Get/1 -> IsPos/1

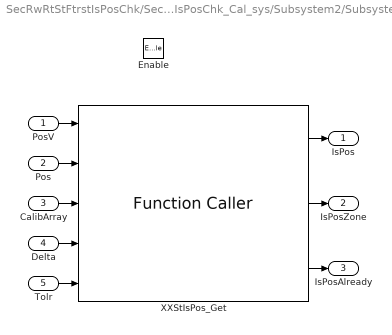
== system SecRwRtStFtrstIsPosChk/SecRwRtStFtrstIsPosChk_Cal_sys/Subsystem2/Subsystem7 ==
  PosV : Inport
  Pos : Inport  Port=2
  CalibArray : Inport  Port=3
  Delta : Inport  Port=4
  Tolr : Inport  Port=5
  Enable : EnablePort
  XXStIsPos_Get : FunctionCaller  FunctionPrototype=[IsPos,IsPosZone,IsPosAlready] = XXStIsPos_Get(PosV,Pos,CalibArray,Delta,Tolr)  InputArgumentSpecifications=boolean(true), uint16(1), uint16([1;1;1]), uint16(1), uint16(1)  OutputArgumentSpecifications=boolean(true), boolean(true), boolean(true)
  IsPos : Outport  VectorParamsAs1DForOutWhenUnconnected=off
  IsPosZone : Outport  Port=2  VectorParamsAs1DForOutWhenUnconnected=off
  IsPosAlready : Outport  Port=3  VectorParamsAs1DForOutWhenUnconnected=off
  wires:
  XXStIsPos_Get/1 -> IsPos/1
  CalibArray/1 -> XXStIsPos_Get/3
  Pos/1 -> XXStIsPos_Get/2
  PosV/1 -> XXStIsPos_Get/1
  XXStIsPos_Get/2 -> IsPosZone/1
  XXStIsPos_Get/3 -> IsPosAlready/1
  Tolr/1 -> XXStIsPos_Get/5
  Delta/1 -> XXStIsPos_Get/4

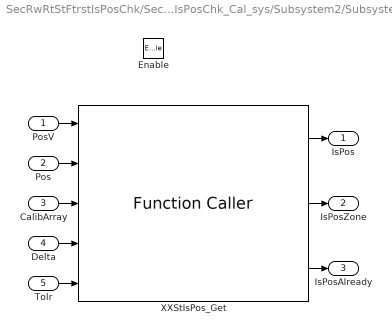
== system SecRwRtStFtrstIsPosChk/SecRwRtStFtrstIsPosChk_Cal_sys/Subsystem2/Subsystem8 ==
  PosV : Inport
  Pos : Inport  Port=2
  CalibArray : Inport  Port=3
  Delta : Inport  Port=4
  Tolr : Inport  Port=5
  Enable : EnablePort
  XXStIsPos_Get : FunctionCaller  FunctionPrototype=[IsPos,IsPosZone,IsPosAlready] = XXStIsPos_Get(PosV,Pos,CalibArray,Delta,Tolr)  InputArgumentSpecifications=boolean(true), uint16(1), uint16([1;1;1]), uint16(1), uint16(1)  OutputArgumentSpecifications=boolean(true), boolean(true), boolean(true)
  IsPos : Outport  VectorParamsAs1DForOutWhenUnconnected=off
  IsPosZone : Outport  Port=2  VectorParamsAs1DForOutWhenUnconnected=off
  IsPosAlready : Outport  Port=3  VectorParamsAs1DForOutWhenUnconnected=off
  wires:
  Delta/1 -> XXStIsPos_Get/4
  Tolr/1 -> XXStIsPos_Get/5
  XXStIsPos_Get/3 -> IsPosAlready/1
  XXStIsPos_Get/2 -> IsPosZone/1
  PosV/1 -> XXStIsPos_Get/1
  Pos/1 -> XXStIsPos_Get/2
  CalibArray/1 -> XXStIsPos_Get/3
  XXStIsPos_Get/1 -> IsPos/1
